simulink model "valvelab_v31"  (R2025b)
settings: Solver=FixedStepDiscrete  StartTime=0  StopTime=1800  FixedStep=0.05  RelTol=1e-3
settings Model: Creator=CCanon  LastModifiedBy=CCanon
settings OptimizationCC: BlockReduction=off

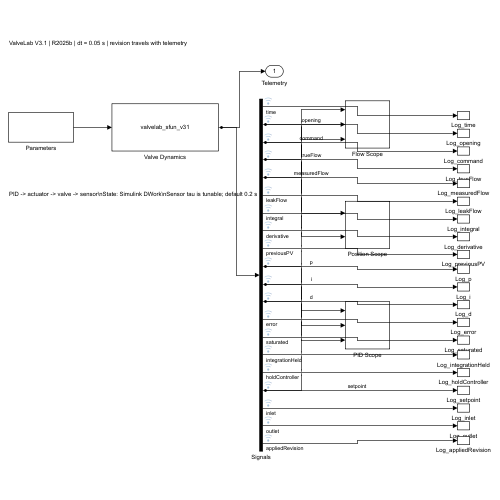
[thumbnail: Simulink's stored preview of the top-level diagram]
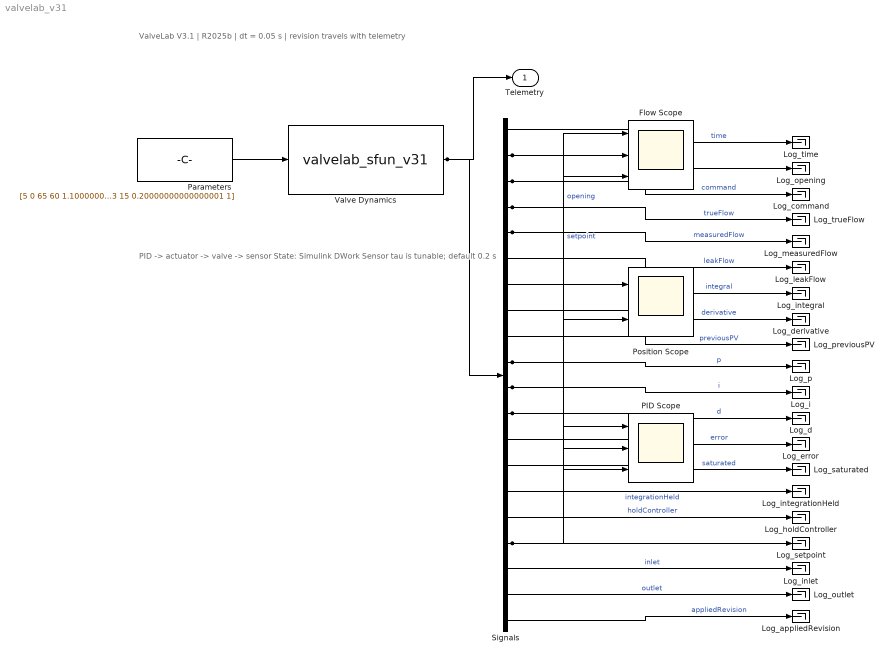
== system valvelab_v31 ==
  note: ValveLab V3.1 | R2025b | dt = 0.05 s | revision travels with telemetry
  note: PID -> actuator -> valve -> sensor\nState: Simulink DWork\nSensor tau is tunable; default 0.2 s
  Flow Scope : Scope  NumInputPorts=3
      settings: TimeSpan=20  Title=SP / Q / PV  YLabel=Flow (L/min)
  Log_appliedRevision : Terminator
  Log_command : Terminator
  Log_d : Terminator
  Log_derivative : Terminator
  Log_error : Terminator
  Log_holdController : Terminator
  Log_i : Terminator
  Log_inlet : Terminator
  Log_integral : Terminator
  Log_integrationHeld : Terminator
  Log_leakFlow : Terminator
  Log_measuredFlow : Terminator
  Log_opening : Terminator
  Log_outlet : Terminator
  Log_p : Terminator
  Log_previousPV : Terminator
  Log_saturated : Terminator
  Log_setpoint : Terminator
  Log_time : Terminator
  Log_trueFlow : Terminator
  PID Scope : Scope  NumInputPorts=3
      settings: TimeSpan=20  ActiveDisplayString=3  Title=D  YLabel=Contribution (%)
  Parameters : Constant  Value=[5 0 65 60 1.1000000000000001 0.55000000000000004 0.040000000000000001 0 0.80000000000000004 12 0 2 1 0 0.050000000000000003 15 0.20000000000000001 1]
  Position Scope : Scope  NumInputPorts=2
      settings: TimeSpan=20  Title=command (u) / opening (x)  YLabel=Position (%)
  Signals : Demux  Outputs=20
  Valve Dynamics : M-S-Function  FunctionName=valvelab_sfun_v31  Parameters=[5 0 65 60 1.1000000000000001 0.55000000000000004 0.040000000000000001 0 0.80000000000000004 12 0 2 1 0 0.050000000000000003 15 0.20000000000000001 1]
  Telemetry : Outport
  wires:
  Parameters/1 -> Valve Dynamics/1
  Valve Dynamics/1 -> Telemetry/1, Signals/1
  Signals/1 -> Log_time/1  "time"
  Signals/2 -> Log_opening/1, Position Scope/2  "opening"
  Signals/3 -> Log_command/1, Position Scope/1  "command"
  Signals/4 -> Log_trueFlow/1, Flow Scope/2  "trueFlow"
  Signals/5 -> Log_measuredFlow/1, Flow Scope/3  "measuredFlow"
  Signals/6 -> Log_leakFlow/1  "leakFlow"
  Signals/7 -> Log_integral/1  "integral"
  Signals/8 -> Log_derivative/1  "derivative"
  Signals/9 -> Log_previousPV/1  "previousPV"
  Signals/10 -> Log_p/1, PID Scope/1  "p"
  Signals/11 -> Log_i/1, PID Scope/2  "i"
  Signals/12 -> Log_d/1, PID Scope/3  "d"
  Signals/13 -> Log_error/1  "error"
  Signals/14 -> Log_saturated/1  "saturated"
  Signals/15 -> Log_integrationHeld/1  "integrationHeld"
  Signals/16 -> Log_holdController/1  "holdController"
  Signals/17 -> Log_setpoint/1, Flow Scope/1  "setpoint"
  Signals/18 -> Log_inlet/1  "inlet"
  Signals/19 -> Log_outlet/1  "outlet"
  Signals/20 -> Log_appliedRevision/1  "appliedRevision"
